simulink model "door_lock_system_testing"  (R2020a)
settings: Solver=FixedStepDiscrete  StartTime=0.0  StopTime=10.0  FixedStep=1  RelTol=1e-3
undefined symbols (not defined in the file or in its folder): carlight, doorlockstatus, DWORK0, DWORK1, sigbuilder_block
libraries: simulink x4
settings Model: Creator=Pravin  LastModifiedBy=hp
settings ConfigComp: CovMetricSettings=dcmwe

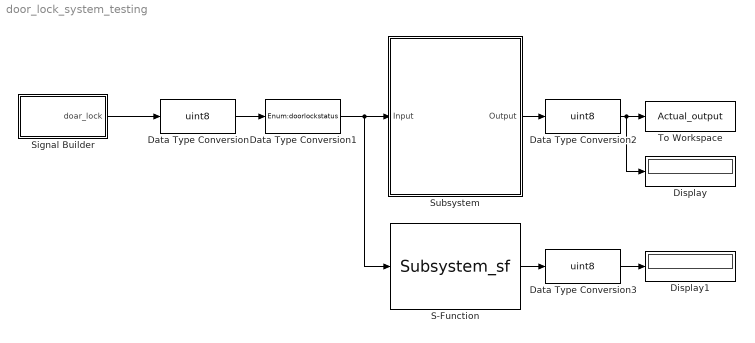
== system door_lock_system_testing ==
  Data Type Conversion : DataTypeConversion  OutDataTypeStr=uint8  SaturateOnIntegerOverflow=on
  Data Type Conversion1 : DataTypeConversion  OutDataTypeStr=Enum:doorlockstatus  SaturateOnIntegerOverflow=on
  Data Type Conversion2 : DataTypeConversion  OutDataTypeStr=uint8  SaturateOnIntegerOverflow=on
  Data Type Conversion3 : DataTypeConversion  OutDataTypeStr=uint8  SaturateOnIntegerOverflow=on
  Display : Display
  Display1 : Display
  S-Function : S-Function  FunctionName=Subsystem_sf  SFunctionDeploymentMode=off  EnableBusSupport=off  SFcnStateName=DWORK0,DWORK1
      settings: SFcnIsStateOwnerBlock=on
  Signal Builder : Subsystem  Tag=STV Subsys  LoadFcn=sigbuilder_block('load');  StartFcn=sigbuilder_block('start');  StopFcn=sigbuilder_block('stop');  ClipboardFcn=sigbuilder_block('clipboard');  mask(Sigbuilder block){tuvar=[0:10]}
      mask help: Simulink:masks:SigbuilderBlock_MD
      mask init:
      | if ~strcmp(get_param(bdroot(gcbh),'SimulationStatus'),'stopped') tuvar = sigbuilder_block('maskInit'); end
      settings: CopyFcn=sigbuilder_block('copy');  DeleteFcn=sigbuilder_block('delete');  ModelCloseFcn=sigbuilder_block('modelClose');  PreSaveFcn=sigbuilder_block('preSave');  PauseFcn=sigbuilder_block('pause');  ContinueFcn=sigbuilder_block('continue');  NameChangeFcn=sigbuilder_block('namechange');  OpenFcn=sigbuilder_block('open',[437.6 153 550.4 359.25 ]);  CloseFcn=sigbuilder_block('close');
      mask Display: plot(0, 0, 100, 100,[2, 2, 32, 32, 2], [68, 8, 8, 68, 68],[32, 2], [38, 38], [32, 19, 2],[53, 60, 44], [32, 17, 17, 2],[16, 16, 31, 31]);txt = getActiveGroup(gcbh);text(2, 100, txt,'verticalAlignment', 'top');
  Subsystem : Subsystem  TreatAsAtomicUnit=on
  To Workspace : ToWorkspace  VariableName=Actual_output  SaveFormat=Timeseries  SampleTime=-1
  wires:
  Signal Builder/1(doar_lock) -> Data Type Conversion/1
  Subsystem/1(Output) -> Data Type Conversion2/1
  Data Type Conversion/1 -> Data Type Conversion1/1
  Data Type Conversion1/1 -> S-Function/1, Subsystem/1(Input)
  S-Function/1 -> Data Type Conversion3/1
  Data Type Conversion2/1 -> Display/1, To Workspace/1
  Data Type Conversion3/1 -> Display1/1

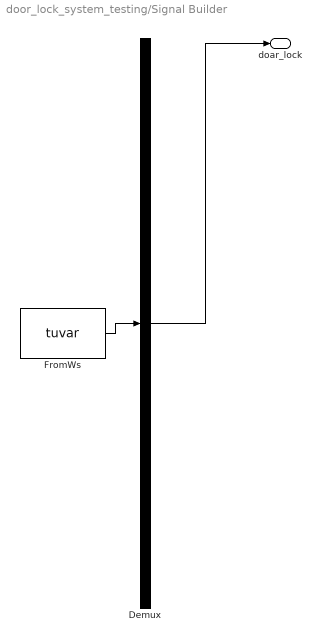
== system door_lock_system_testing/Signal Builder ==
  Demux : Demux  Tag=STV Demux  Outputs=1
      settings: DisplayOption=none
  FromWs : FromWorkspace  Tag=STV FromWs  VariableName=tuvar
      SigBuilderData=|
      | common.afterFinalStr = 'Extrapolate'
      | common.sampleTime = 0
      | dataSet.timeRange = [0 10]
      | dataSet.name = 'Sheet1'
      | sbobj.Groups.Name = 'Sheet1'
      | sbobj.Groups.Signals.Name = 'doar_lock'
      | sbobj.Groups.Signals.XData = [0 1 2 3 4 5 6 7 8 9 10]
      | sbobj.Groups.Signals.YData = [1 1 0 1 0 1 1 1 1 1 0]
  doar_lock : Outport  Tag=STV Outport
  wires:
  Demux/1 -> doar_lock/1
  FromWs/1 -> Demux/1

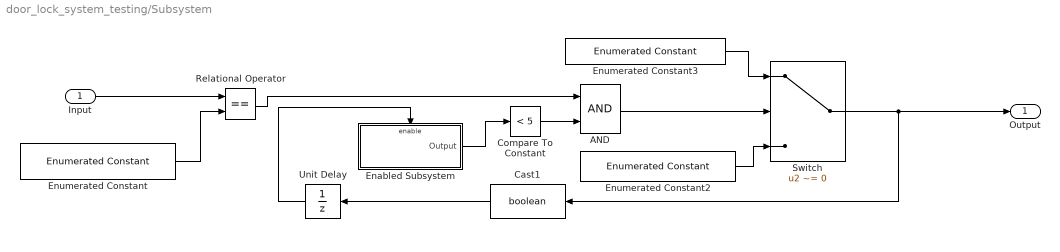
== system door_lock_system_testing/Subsystem ==
  Input : Inport
  AND : Logic  AllPortsSameDT=off  OutDataTypeStr=boolean
  Cast1 : DataTypeConversion  OutDataTypeStr=boolean
  Compare To Constant : simulink/Logic and Bit Operations/Compare To Constant  relop=<  const=5  OutDataTypeStr=boolean
  Enabled Subsystem : Subsystem  TreatAsAtomicUnit=on
  Enumerated Constant : simulink/Sources/Enumerated Constant  OutDataTypeStr=Enum: doorlockstatus  Value=doorlockstatus.door_lock_close  SampleTime=inf
  Enumerated Constant2 : simulink/Sources/Enumerated Constant  OutDataTypeStr=Enum: carlight  Value=carlight.Head_light_tail_light_off  SampleTime=inf
  Enumerated Constant3 : simulink/Sources/Enumerated Constant  OutDataTypeStr=Enum: carlight  Value=carlight.Head_light_tail_light_on  SampleTime=inf
  Relational Operator : RelationalOperator  Operator===  OutDataTypeStr=boolean  RndMeth=Simplest
  Switch : Switch  Criteria=u2 ~= 0
  Unit Delay : UnitDelay  SampleTime=-1  HasFrameUpgradeWarning=on
  Output : Outport
  wires:
  AND/1 -> Switch/2
  Enumerated Constant/1 -> Relational Operator/2
  Switch/1 -> Output/1, Cast1/1
  Relational Operator/1 -> AND/1
  Unit Delay/1 -> Enabled Subsystem/Enable
  Enabled Subsystem/1(Output) -> Compare To Constant/1
  Enumerated Constant3/1 -> Switch/1
  Cast1/1 -> Unit Delay/1
  Compare To Constant/1 -> AND/2
  Input/1 -> Relational Operator/1
  Enumerated Constant2/1 -> Switch/3

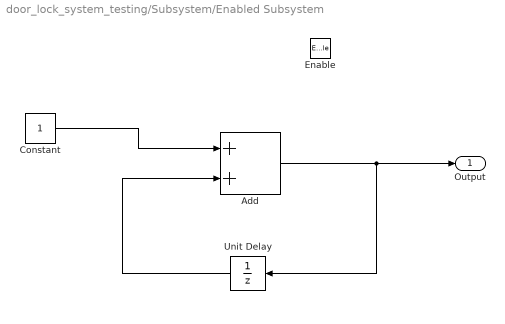
== system door_lock_system_testing/Subsystem/Enabled Subsystem ==
  Enable : EnablePort
  Add : Sum
  Constant : Constant
  Unit Delay : UnitDelay  SampleTime=-1  HasFrameUpgradeWarning=on
  Output : Outport  VectorParamsAs1DForOutWhenUnconnected=off
  wires:
  Add/1 -> Output/1, Unit Delay/1
  Constant/1 -> Add/1
  Unit Delay/1 -> Add/2
